simulink model "Top_Level"  (R2022a)
settings: Solver=VariableStepAuto  StartTime=0.0  StopTime=10.0  RelTol=1e-3
settings Model: Creator=joedo  LastModifiedBy=joedo

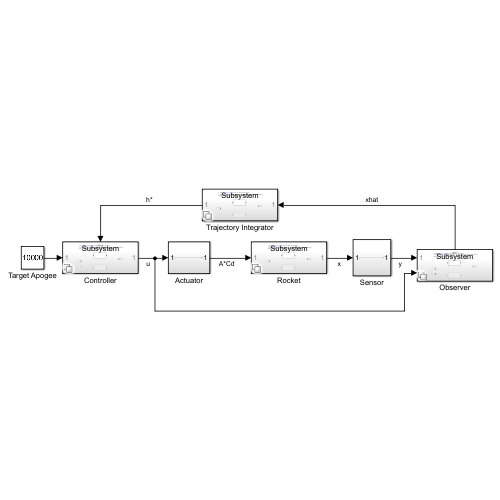
[thumbnail: Simulink's stored preview of the top-level diagram]
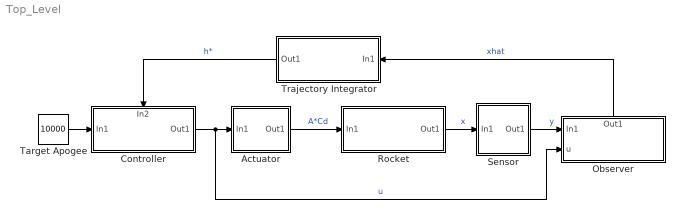
== system Top_Level ==
  Actuator : Subsystem
  Controller : Subsystem  Variant=on
      settings: PortSchema="{\"entries\":[{\"content\":{\"sides\":[{\"content\":{\"connectorIds\":[\"In1\"]},\"type\":\"ConnectorPlacement.EquallySpacedRectSide\",\"uuid\":\"67748641-5e06-41a3-bf22-d2b4fd99d06e\"},{\"content\":{\"connectorIds\":[\"Out1\"],\"side\":\"RIGHT\"},\"type\":\"ConnectorPlacement.EquallySpacedRectSide\",\"uuid\":\"75f1e930-e584-4d04-8d12-ea7ab32aa1fb\"},{\"content\":{\"connectorIds\":[\"In2\"],\"side\":\"TOP\"},\"type\":\"ConnectorPlacement.EquallySpacedRectSide\",\"uuid\":\"417ddf59-a249-4509-a718-811260073461\"}]},\"type\":\"ConnectorPlacement.EquallySpacedConnector\",\"uuid\":\"eeb0d859-6383-43e6-84fe-9dd5f9014128\"}],\"packageUris\":[\"http://schema.mathworks.com/mf0/Connector/R2020b\"],\"version\":\"1.0\"}"
  Observer : Subsystem  Variant=on
      settings: PortSchema="{\"entries\":[{\"content\":{\"sides\":[{\"content\":{\"connectorIds\":[\"In1\",\"In2\"]},\"type\":\"ConnectorPlacement.EquallySpacedRectSide\",\"uuid\":\"67748641-5e06-41a3-bf22-d2b4fd99d06e\"},{\"content\":{\"connectorIds\":[],\"side\":\"RIGHT\"},\"type\":\"ConnectorPlacement.EquallySpacedRectSide\",\"uuid\":\"75f1e930-e584-4d04-8d12-ea7ab32aa1fb\"},{\"content\":{\"connectorIds\":[\"Out1\"],\"side\":\"TOP\"},\"type\":\"ConnectorPlacement.EquallySpacedRectSide\",\"uuid\":\"417ddf59-a249-4509-a718-811260073461\"}]},\"type\":\"ConnectorPlacement.EquallySpacedConnector\",\"uuid\":\"eeb0d859-6383-43e6-84fe-9dd5f9014128\"}],\"packageUris\":[\"http://schema.mathworks.com/mf0/Connector/R2020b\"],\"version\":\"1.0\"}"
  Rocket : Subsystem  Variant=on
  Sensor : Subsystem
  Target Apogee : Constant  Value=10000
  Trajectory Integrator : Subsystem  Variant=on
      settings: PortSchema="{\"entries\":[{\"content\":{\"sides\":[{\"content\":{\"connectorIds\":[\"Out1\"]},\"type\":\"ConnectorPlacement.EquallySpacedRectSide\",\"uuid\":\"67748641-5e06-41a3-bf22-d2b4fd99d06e\"},{\"content\":{\"connectorIds\":[\"In1\"],\"side\":\"RIGHT\"},\"type\":\"ConnectorPlacement.EquallySpacedRectSide\",\"uuid\":\"75f1e930-e584-4d04-8d12-ea7ab32aa1fb\"},{\"content\":{\"connectorIds\":[],\"side\":\"TOP\"},\"type\":\"ConnectorPlacement.EquallySpacedRectSide\",\"uuid\":\"417ddf59-a249-4509-a718-811260073461\"}]},\"type\":\"ConnectorPlacement.EquallySpacedConnector\",\"uuid\":\"eeb0d859-6383-43e6-84fe-9dd5f9014128\"}],\"packageUris\":[\"http://schema.mathworks.com/mf0/Connector/R2020b\"],\"version\":\"1.0\"}"
  wires:
  Controller/1(Out1) -> Observer/2(u), Actuator/1(In1)  "u"
  Actuator/1(Out1) -> Rocket/1(In1)  "A*Cd"
  Target Apogee/1 -> Controller/1(In1)
  Rocket/1(Out1) -> Sensor/1(In1)  "x"
  Observer/1(Out1) -> Trajectory Integrator/1(In1)  "xhat"
  Trajectory Integrator/1(Out1) -> Controller/2(In2)  "h*"
  Sensor/1(Out1) -> Observer/1(In1)  "y"

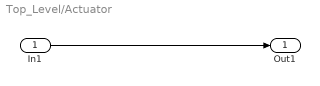
== system Top_Level/Actuator ==
  In1 : Inport
  Out1 : Outport
  wires:
  In1/1 -> Out1/1

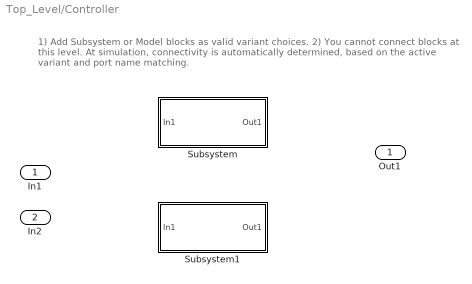
== system Top_Level/Controller ==
  note: 1) Add Subsystem or Model blocks as valid variant choices.
      | 2) You cannot connect blocks at this level. At simulation, connectivity is automatically
      | determined, based on the active variant and port name matching.
  In1 : Inport
  In2 : Inport  Port=2
  Subsystem : Subsystem  VariantControl=true
  Subsystem1 : Subsystem  VariantControl=false
  Out1 : Outport

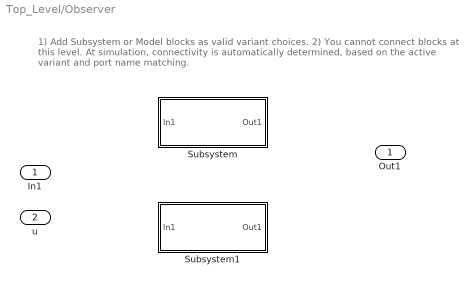
== system Top_Level/Observer ==
  note: 1) Add Subsystem or Model blocks as valid variant choices.
      | 2) You cannot connect blocks at this level. At simulation, connectivity is automatically
      | determined, based on the active variant and port name matching.
  In1 : Inport
  u : Inport  Port=2
  Subsystem : Subsystem  VariantControl=true
  Subsystem1 : Subsystem  VariantControl=false
  Out1 : Outport

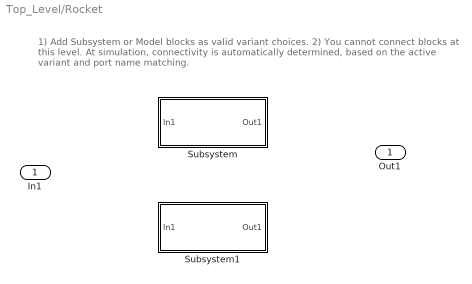
== system Top_Level/Rocket ==
  note: 1) Add Subsystem or Model blocks as valid variant choices.
      | 2) You cannot connect blocks at this level. At simulation, connectivity is automatically
      | determined, based on the active variant and port name matching.
  In1 : Inport
  Subsystem : Subsystem  VariantControl=true
  Subsystem1 : Subsystem  VariantControl=false
  Out1 : Outport

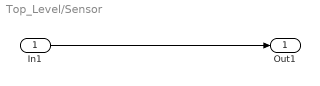
== system Top_Level/Sensor ==
  In1 : Inport
  Out1 : Outport
  wires:
  In1/1 -> Out1/1

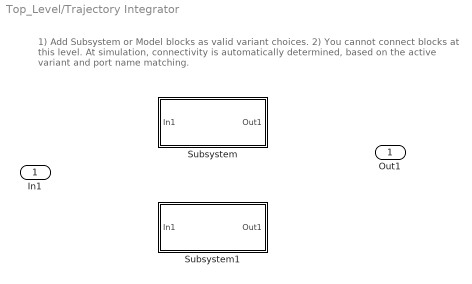
== system Top_Level/Trajectory Integrator ==
  note: 1) Add Subsystem or Model blocks as valid variant choices.
      | 2) You cannot connect blocks at this level. At simulation, connectivity is automatically
      | determined, based on the active variant and port name matching.
  In1 : Inport
  Subsystem : Subsystem  VariantControl=true
  Subsystem1 : Subsystem  VariantControl=false
  Out1 : Outport

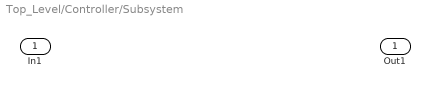
== system Top_Level/Controller/Subsystem ==
  In1 : Inport
  Out1 : Outport

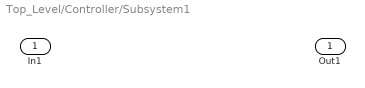
== system Top_Level/Controller/Subsystem1 ==
  In1 : Inport
  Out1 : Outport

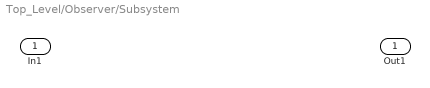
== system Top_Level/Observer/Subsystem ==
  In1 : Inport
  Out1 : Outport

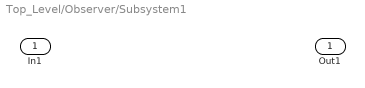
== system Top_Level/Observer/Subsystem1 ==
  In1 : Inport
  Out1 : Outport

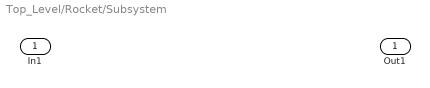
== system Top_Level/Rocket/Subsystem ==
  In1 : Inport
  Out1 : Outport

== system Top_Level/Rocket/Subsystem1 ==
  In1 : Inport
  Out1 : Outport

== system Top_Level/Trajectory Integrator/Subsystem ==
  In1 : Inport
  Out1 : Outport

== system Top_Level/Trajectory Integrator/Subsystem1 ==
  In1 : Inport
  Out1 : Outport
